simulink model "Boat_NonLinear"  (R2020a)
settings: Solver=VariableStepAuto  StartTime=0.0  StopTime=50  MaxStep=0.001  RelTol=1e-3
settings Model: NumberOfSteps=10  Creator=micro microndas  LastModifiedBy=micro microndas

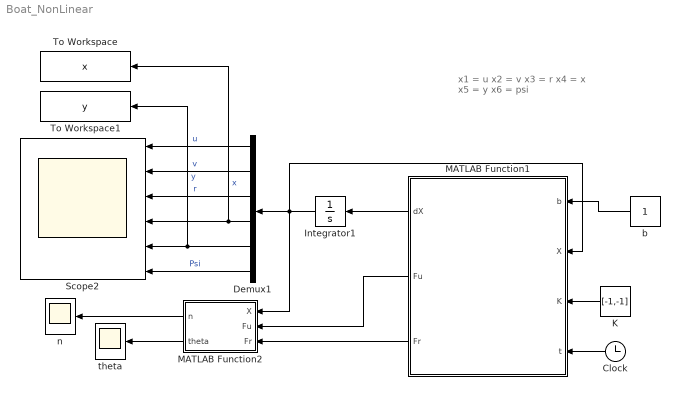
== system Boat_NonLinear ==
  note: x1 = u
      | x2 = v
      | x3 = r
      | x4 = x
      | x5 = y
      | x6 = psi
  Clock : Clock
  Demux1 : Demux  Outputs=6
  Integrator1 : Integrator  InitialCondition=[0 0 0 0 0 pi/4]
  K : Constant  Value=[-1,-1]
  MATLAB Function1 : MATLAB Function  TreatAsAtomicUnit=on
  MATLAB Function2 : MATLAB Function  TreatAsAtomicUnit=on
  Scope2 : Scope  NumInputPorts=6
  To Workspace : ToWorkspace  VariableName=x  SampleTime=-1
      settings: Save2DSignal=2-D array (concatenate along first dimension)
  To Workspace1 : ToWorkspace  VariableName=y  SampleTime=-1
      settings: Save2DSignal=2-D array (concatenate along first dimension)
  b : Constant
  n : Scope
  theta : Scope
  wires:
  MATLAB Function1/1(dX) -> Integrator1/1
  b/1 -> MATLAB Function1/1(b)
  K/1 -> MATLAB Function1/3(K)
  Integrator1/1 -> MATLAB Function1/2(X), MATLAB Function2/1(X), Demux1/1
  Demux1/1 -> Scope2/1  "u"
  Demux1/2 -> Scope2/2  "v"
  Demux1/3 -> Scope2/3  "r"
  Demux1/4 -> To Workspace/1, Scope2/4  "x"
  Demux1/5 -> To Workspace1/1, Scope2/5  "y"
  Demux1/6 -> Scope2/6  "Psi"
  MATLAB Function1/3(Fr) -> MATLAB Function2/3(Fr)
  MATLAB Function1/2(Fu) -> MATLAB Function2/2(Fu)
  MATLAB Function2/2(theta) -> theta/1
  Clock/1 -> MATLAB Function1/4(t)
  MATLAB Function2/1(n) -> n/1

== matlab function Boat_NonLinear/MATLAB Function1 ==
  data: b input; X input; dX output; K input; Fu output; Fr output; t input
function [dX,Fu, Fr] = fcn(b, X, K, t)

k1 = K(1);
k2 = K(2);

x5_ref = 50+20*sin(0.1*t);
x4_ref = 50+20*cos(0.1*t);

dx5_ref = 20*0.1*cos(0.1*t);
dx4_ref = -20*0.1*sin(0.1*t);

ddx5_ref = -20*0.1*0.1*sin(0.1*t);
ddx4_ref = -20*0.1*0.1*cos(0.1*t);

e1 =  [x4_ref;
       x5_ref] - [X(4);
                  X(5)];
d_e1 = [dx4_ref; 
        dx5_ref ] - [ cos(X(6)), -sin(X(6)); 
                      sin(X(6)), cos(X(6))]*[X(1);X(2)];

x_ref = [ cos(X(6)), sin(X(6));
             -sin(X(6)), cos(X(6))]*(  [dx4_ref; 
                                        dx5_ref ]  - k1*e1);

dx_ref = [ -sin(X(6)), cos(X(6));
              -cos(X(6)), -sin(X(6))]*( [dx4_ref; 
                                         dx5_ref ] -e1*k1 ) + [ cos(X(6)), sin(X(6));
                                                               -sin(X(6)), cos(X(6))]*( [ddx4_ref;
                                                                                         ddx5_ref] -d_e1*k1 );
e2 = [x_ref(1);
      x_ref(2)] - [X(1);
                 X(2)];
             
u = inv([0.0185, 0;
            0, 0.0110*b])*( [dx_ref(1);
                             dx_ref(2)] - [-0.2775, 0;
                                         0.7*X(3), 0.2083]*[X(1);
                                                            X(2)] -e2*k2 );
dX = [-0.2775*X(1);0.7*X(1)*X(3) + 0.2083*X(2);0.7*X(1)*X(3) + 0.2083*X(2);X(1)*cos(X(6))-X(2)*sin(X(6));X(1)*sin(X(6)) + X(2)*cos(X(6));X(3)] + [[0.0185, 0;0,0.011*b];0, 0.011*b;0, 0;0, 0;0, 0]*u;

Fu = u(1);
Fr = u(2);

== matlab function Boat_NonLinear/MATLAB Function2 ==
  data: X input; Fu input; n output; Fr input; theta output
function [n, theta] = fcn(X, Fu, Fr)

T1 = 0.26;  T2= 0.1; b = 1; 

V = sqrt( X(1)^2 + (X(3)*b)^2 );
F = sqrt( Fu^2 + Fr^2 ); 

theta = atan(-Fr/Fu);
n =( T1*V + sqrt( (T2*V)^2 + 4*F*T2)) / (2*T1^2);
